simulink model "LateralDynamics"  (R2014a)
settings: Solver=ode45  StartTime=0.0  StopTime=10.0  RelTol=1e-3
values from neighbouring files (symbols this model uses):
  a_phi1 = -.5*rho*Va^2*S*b*C_pp*b/(2*Va)    (= 29.79115125)    [MAIN.m]
  a_phi2 = .5*rho*Va^2*S*b*C_pdeltaA    (= 80.9375)    [MAIN.m]
  g = 9.81    [MAIN.m]    (also in MAINLongitudinal.m)
  kd_phi = (2*zeta_phi*w_nphi-a_phi1)/a_phi2    [MAIN.m]
  ki_X = wn_X^2*Vg/g    [MAIN.m]
  kp_phi = deltaa_max/e_phimax*sign(a_phi1)    [MAIN.m]
  kp_X = 2*zeta_X*wn_X*Vg/g    [MAIN.m]
  Vg = 15    [MAIN.m]    (also in MAINLongitudinal.m = 10)
settings Model: Creator=Nathan  LastModifiedBy=Nathan

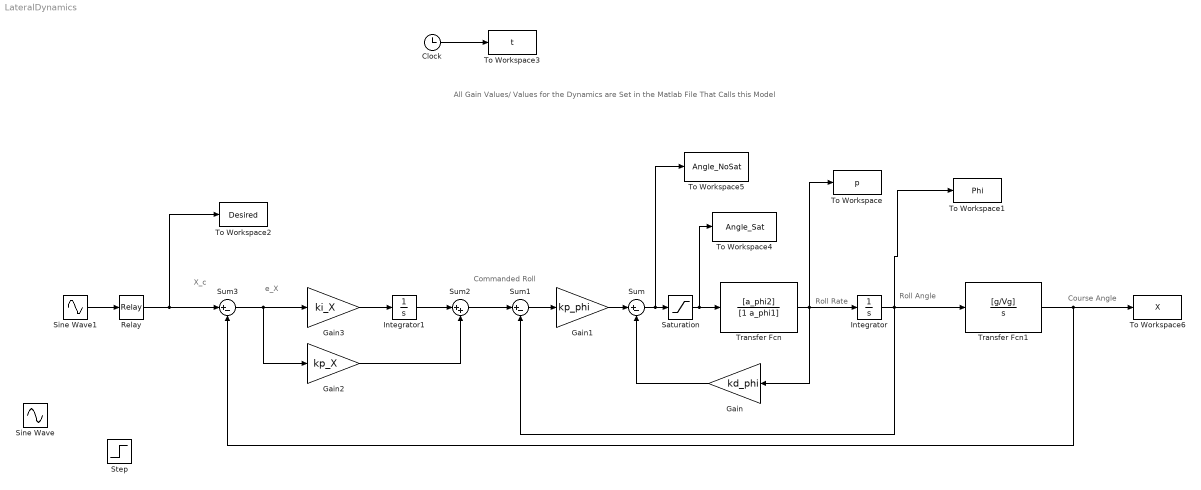
== system LateralDynamics ==
  note: e_X
  note: X_c
  note: Commanded Roll
  note: Course Angle
  note: All Gain Values/ Values for the Dynamics are Set in the Matlab File That Calls this Model
  note: Roll Rate
  note: Roll Angle
  Clock : Clock
  Gain : Gain  Gain=kd_phi
  Gain1 : Gain  Gain=kp_phi
  Gain2 : Gain  Gain=kp_X
  Gain3 : Gain  Gain=ki_X
  Integrator : Integrator
  Integrator1 : Integrator
  Relay : Relay  OffOutputValue=-1
  Saturation : Saturate  UpperLimit=1000  LowerLimit=-1000  LinearizeAsGain=off  ZeroCross=off
  Sine Wave : Sin  SampleTime=0
  Sine Wave1 : Sin  SampleTime=0
  Step : Step  Time=2  SampleTime=0
  Sum : Sum  Inputs=|+-
  Sum1 : Sum  Inputs=|+-
  Sum2 : Sum  Inputs=|++
  Sum3 : Sum  Inputs=|+-
  To Workspace : ToWorkspace  VariableName=p  SampleTime=-1
  To Workspace1 : ToWorkspace  VariableName=Phi  SampleTime=-1
  To Workspace2 : ToWorkspace  VariableName=Desired  SampleTime=-1
  To Workspace3 : ToWorkspace  VariableName=t  SampleTime=-1
  To Workspace4 : ToWorkspace  VariableName=Angle_Sat  SampleTime=-1
  To Workspace5 : ToWorkspace  VariableName=Angle_NoSat  SampleTime=-1
  To Workspace6 : ToWorkspace  VariableName=X  SampleTime=-1
  Transfer Fcn : TransferFcn  Numerator=[a_phi2]  Denominator=[1 a_phi1]
  Transfer Fcn1 : TransferFcn  Numerator=[g/Vg]  Denominator=[1 0]
  wires:
  Gain/1 -> Sum/2
  Sum/1 -> To Workspace5/1, Saturation/1
  Transfer Fcn/1 -> Integrator/1, To Workspace/1, Gain/1
  Integrator/1 -> Transfer Fcn1/1, To Workspace1/1, Sum1/2
  Clock/1 -> To Workspace3/1
  Sine Wave1/1 -> Relay/1
  Saturation/1 -> To Workspace4/1, Transfer Fcn/1
  Sum1/1 -> Gain1/1
  Gain1/1 -> Sum/1
  Integrator1/1 -> Sum2/1
  Sum2/1 -> Sum1/1
  Gain3/1 -> Integrator1/1
  Gain2/1 -> Sum2/2
  Sum3/1 -> Gain3/1, Gain2/1
  Transfer Fcn1/1 -> To Workspace6/1, Sum3/2
  Relay/1 -> To Workspace2/1, Sum3/1
